simulink model "Time_delay_system"  (Simulink 7.6)
settings: Solver=ode45  StartTime=0.0  StopTime=10.0  RelTol=1e-3
settings Model: Creator=administrator  LastModifiedBy=administrator

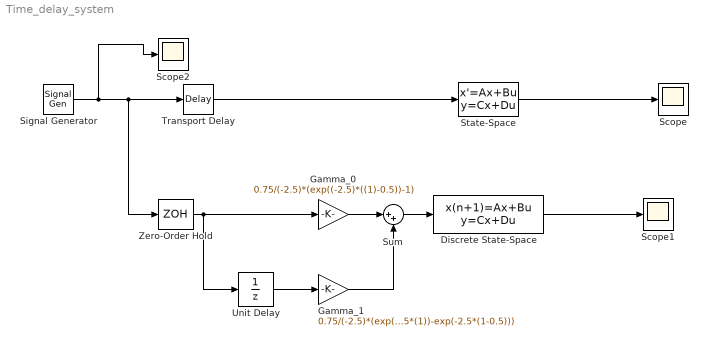
== system Time_delay_system ==
  Discrete State-Space : DiscreteStateSpace  A=expm(-2.5*1)  D=0  SampleTime=-1
  Gamma_0 : Gain  Gain=0.75/(-2.5)*(exp((-2.5)*((1)-0.5))-1)
  Gamma_1 : Gain  Gain=0.75/(-2.5)*(exp(-2.5*(1))-exp(-2.5*(1-0.5)))
  Scope : Scope
  Scope1 : Scope
  Scope2 : Scope
      settings: SaveName=ScopeData2
  Signal Generator : SignalGenerator  WaveForm=square  Frequency=pi  Units=rad/sec
  State-Space : StateSpace  A=-2.5  B=0.75  D=0
  Sum : Sum  Inputs=|++
  Transport Delay : TransportDelay  DelayTime=0.5
  Unit Delay : UnitDelay  SampleTime=-1
  Zero-Order Hold : ZeroOrderHold
  wires:
  Signal Generator/1 -> Transport Delay/1, Zero-Order Hold/1, Scope2/1
  Transport Delay/1 -> State-Space/1
  State-Space/1 -> Scope/1
  Zero-Order Hold/1 -> Unit Delay/1, Gamma_0/1
  Unit Delay/1 -> Gamma_1/1
  Gamma_0/1 -> Sum/1
  Gamma_1/1 -> Sum/2
  Sum/1 -> Discrete State-Space/1
  Discrete State-Space/1 -> Scope1/1
